simulink model "sistemaNonLineare3"  (R2025b)
settings: Solver=VariableStepAuto  StartTime=0.0  StopTime=0.05  RelTol=1e-3
values from neighbouring files (symbols this model uses):
  C_num = double(C_eq)    [codiceProgetto3.m]
  u_e_val = k_val * theta_e_val    (= 52.3598775598)    [codiceProgetto3.m]
  x_e_val = [theta_e_val; 0]    [codiceProgetto3.m]
  y_e_val = theta_e_val    (= 1.0471975512)    [codiceProgetto3.m]
libraries: cstblocks x1
settings Model: Creator=singh  LastModifiedBy=ospite
settings DebuggingCC: UnderspecifiedInitializationDetection=Classic  MergeDetectMultiDrivingBlocksExec=none
settings ModelReferenceCC: PropagateSignalLabelsOutOfModel=off

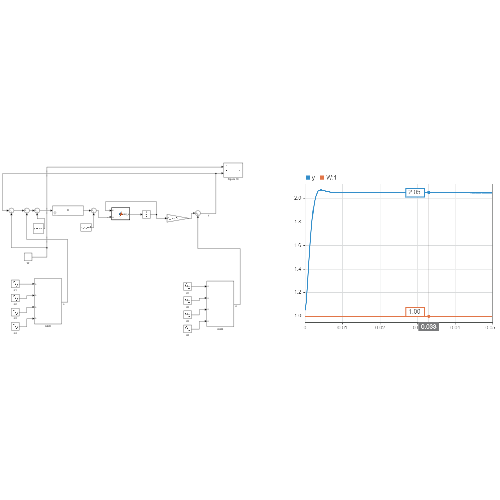
[thumbnail: Simulink's stored preview of the top-level diagram]
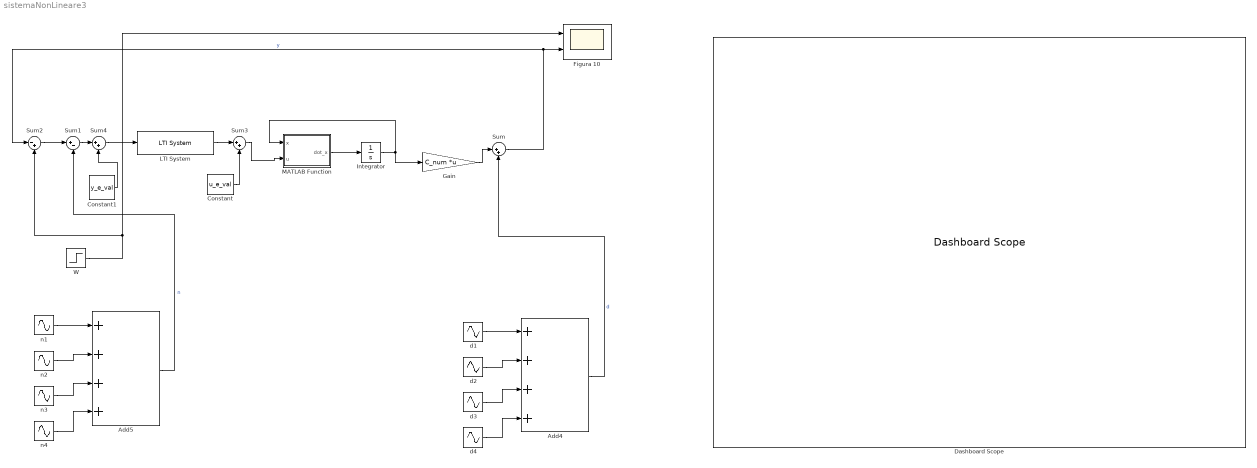
== system sistemaNonLineare3 ==
  Add4 : Sum  Inputs=++++
  Add5 : Sum  Inputs=++++
  Constant : Constant  Value=u_e_val
  Constant1 : Constant  Value=y_e_val
  Dashboard Scope : DashboardScope  Ymin=1  FontColor=[0.0, 0.0, 0.0]
  Figura 10 : Scope  NumInputPorts=2
      settings: ActiveDisplayYMinimum=1.9009131951042531  ActiveDisplayYMaximum=2.0969240709263395  DataLoggingSaveFormat=Array
  Gain : Gain  Gain=C_num  Multiplication=Matrix(K*u)
  Integrator : Integrator  InitialCondition=x_e_val
  LTI System : cstblocks/LTI System  sys=R  IC=[]  PadeOrder=0
  MATLAB Function : MATLAB Function  TreatAsAtomicUnit=on
  Sum : Sum  Inputs=|++
  Sum1 : Sum  Inputs=|+-
  Sum2 : Sum  Inputs=|-+
  Sum3 : Sum  Inputs=|++
  Sum4 : Sum  Inputs=|++
  W : Step  Time=0  SampleTime=0
  d1 : Sin  Frequency=0.1*1  SampleTime=0
  d2 : Sin  Frequency=0.1*2  SampleTime=0
  d3 : Sin  Frequency=0.1*3  SampleTime=0
  d4 : Sin  Frequency=0.1*4  SampleTime=0
  n1 : Sin  Frequency=50000*1  SampleTime=0
  n2 : Sin  Frequency=50000*2  SampleTime=0
  n3 : Sin  Frequency=50000*3  SampleTime=0
  n4 : Sin  Frequency=50000*4  SampleTime=0
  wires:
  Add4/1 -> Sum/2  "d"
  LTI System/1 -> Sum3/1
  Constant1/1 -> Sum4/2
  n2/1 -> Add5/2
  W/1 -> Sum2/2, Figura 10/1
  n4/1 -> Add5/4
  Sum2/1 -> Sum1/1
  Sum4/1 -> LTI System/1
  d1/1 -> Add4/1
  Sum/1 -> Sum2/1, Figura 10/2  "y"
  d3/1 -> Add4/3
  Constant/1 -> Sum3/2
  n3/1 -> Add5/3
  d2/1 -> Add4/2
  d4/1 -> Add4/4
  Add5/1 -> Sum1/2  "n"
  Sum1/1 -> Sum4/1
  n1/1 -> Add5/1
  Sum3/1 -> MATLAB Function/2(u)
  MATLAB Function/1(dot_x) -> Integrator/1
  Integrator/1 -> Gain/1, MATLAB Function/1(x)
  Gain/1 -> Sum/1

== matlab function sistemaNonLineare3/MATLAB Function ==
  data: x input; u input; dot_x output
function dot_x = fcn(x,u)

%valori numerici tratti dalle specifiche
k_val=50;
beta_val=1;

dot_x = zeros(2,1);

dot_x(1) = x(2);
dot_x(2) = (u - beta_val*x(2) - k_val*x(1)) / (1.7+ (0.1*cos(1*pi/3 -0.04)) + (0.7*cos(2*pi/3 + 2.9)) + (0.09*cos(3*pi/3 + 2.8)) + (0.02*cos(4*pi/3-2.6)));
dot_x = [dot_x(1); dot_x(2)];
